simulink model "CNL_TP1_SysLinSat_SimuLink_Q1CIm10m10_edita"  (R2018a)
settings: Solver=VariableStepAuto  StartTime=0.0  StopTime=10.0  RelTol=1e-3
settings Model: Creator=tunn  LastModifiedBy=tunn

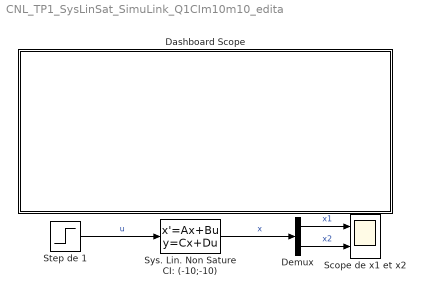
== system CNL_TP1_SysLinSat_SimuLink_Q1CIm10m10_edita ==
  " Sys. Lin. Non Sature CI: (-10;-10)" : StateSpace  A=[0 1; -1 -1]  B=[0; 0]  C=eye(2)  D=[0; 0]  InitialCondition=-10
  Dashboard Scope : Subsystem  DialogController=hmiCreateDDGDialog  IsWebBlock=on  mask(MWDashboardBlock){webBlockId=6d8d5469-bd37-4983-a92c-f3284b4fdc4c, webBlockType=sdiscope, ShowInitialText=on, HMISrcModelName=untitled}
      mask prompts: webBlockId "WebBlock Id"; webBlockType "WebBlock Type"; HMISrcModelName "Source Model"
      mask help: SimulinkHMI:dialogs:HMIScopeDialogDesc
      mask Help: helpview([docroot '/mapfiles/simulink.map'], 'hmi_scope')
      mask Display:
      | if strcmp(get_param(bdroot(gcb),'BlockDiagramType'), 'library')
      |     image([(matlabroot) '/toolbox/simulink/hmi/icons/DashboardScope.png']);
      | end
  Demux : Demux  Outputs=2
  Scope de x1 et x2 : Scope  NumInputPorts=2
  Step de 1 : Step  Time=0  SampleTime=0
  wires:
  " Sys. Lin. Non Sature CI: (-10;-10)"/1 -> Demux/1  "x"
  Step de 1/1 -> " Sys. Lin. Non Sature CI: (-10;-10)"/1  "u"
  Demux/2 -> Scope de x1 et x2/2  "x2"
  Demux/1 -> Scope de x1 et x2/1  "x1"

== system CNL_TP1_SysLinSat_SimuLink_Q1CIm10m10_edita/Dashboard Scope ==
